simulink model "Lab8"  (R2022b)
settings: Solver=ode1  StartTime=0.0  StopTime=300  FixedStep=0.01  RelTol=1e-3
values from neighbouring files (symbols this model uses):
  Ap = 2.5    [Lab08.m]
  As = 0.1    [Lab08.m]
  fp = 0.2    [Lab08.m]
  fs = 0.015    [Lab08.m]
  Kp = 6    [Lab08.m]
  Ks = 1    [Lab08.m]
libraries: simulink x1, simulink_extras x1
settings Model: Creator=Wasif  LastModifiedBy=Wasif
settings DataIOCC: ReturnWorkspaceOutputs=off

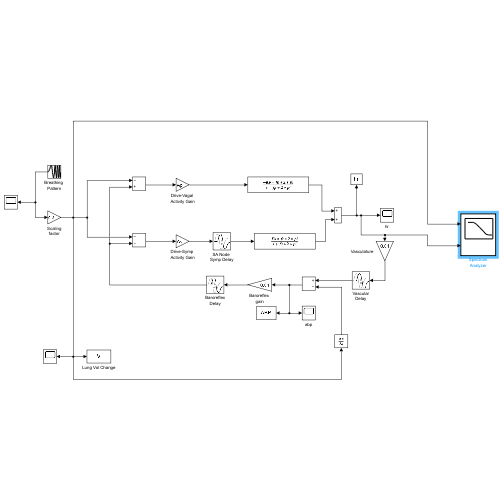
[thumbnail: Simulink's stored preview of the top-level diagram]
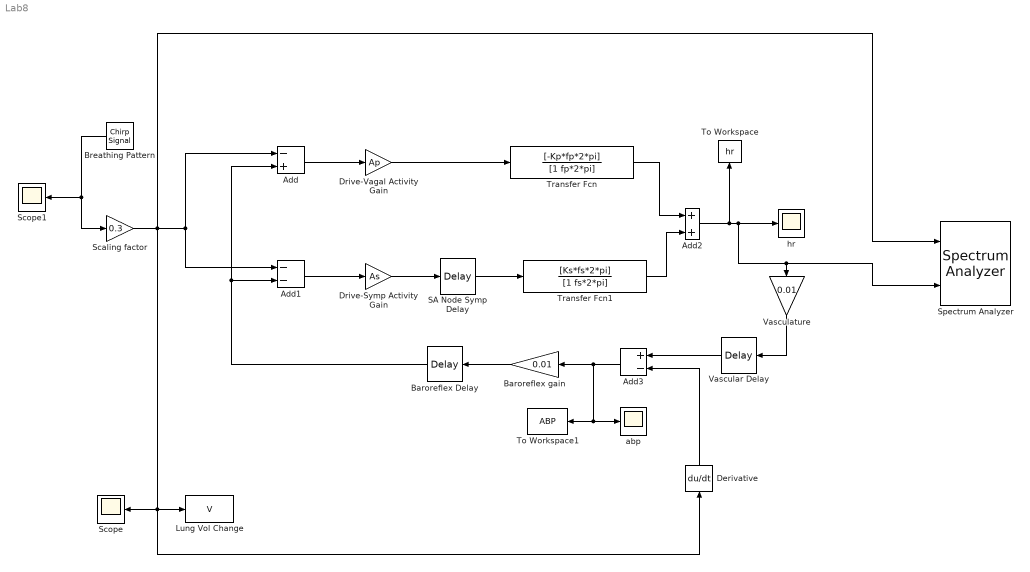
== system Lab8 ==
  Add : Sum  Inputs=-+
  Add1 : Sum  Inputs=--
  Add2 : Sum
  Add3 : Sum  Inputs=+-
  Baroreflex Delay : TransportDelay  DelayTime=0.3
  Baroreflex gain : Gain  Gain=0.01
  Breathing Pattern : simulink/Sources/Chirp Signal  f1=0.005  T=300  f2=0.5
  Derivative : Derivative
  Drive-Symp Activity Gain : Gain  Gain=As
  Drive-Vagal Activity Gain : Gain  Gain=Ap
  Lung Vol Change : ToWorkspace  VariableName=V  SampleTime=-1
  SA Node Symp Delay : TransportDelay  DelayTime=1.7
  Scaling factor : Gain  Gain=0.3
  Scope : Scope
  Scope1 : Scope
  Spectrum Analyzer : simulink_extras/Additional Sinks/Spectrum Analyzer  npts=256  fftpts=256  HowOften=64  sampleT=0.1
  To Workspace : ToWorkspace  VariableName=hr  SampleTime=-1
  To Workspace1 : ToWorkspace  VariableName=ABP  SampleTime=-1
  Transfer Fcn : TransferFcn  Numerator=[-Kp*fp*2*pi]  Denominator=[1 fp*2*pi]
  Transfer Fcn1 : TransferFcn  Numerator=[Ks*fs*2*pi]  Denominator=[1 fs*2*pi]
  Vascular Delay : TransportDelay  DelayTime=0.44
  Vasculature : Gain  Gain=0.01
  abp : Scope
  hr : Scope
  wires:
  Breathing Pattern/1 -> Scope1/1, Scaling factor/1
  Scaling factor/1 -> Derivative/1, Scope/1, Lung Vol Change/1, Spectrum Analyzer/1, Add/1, Add1/1
  Add/1 -> Drive-Vagal Activity Gain/1
  Add1/1 -> Drive-Symp Activity Gain/1
  Drive-Symp Activity Gain/1 -> SA Node Symp Delay/1
  Drive-Vagal Activity Gain/1 -> Transfer Fcn/1
  SA Node Symp Delay/1 -> Transfer Fcn1/1
  Transfer Fcn/1 -> Add2/1
  Transfer Fcn1/1 -> Add2/2
  Add2/1 -> To Workspace/1, Spectrum Analyzer/2, Vasculature/1, hr/1
  Vasculature/1 -> Vascular Delay/1
  Vascular Delay/1 -> Add3/1
  Add3/1 -> abp/1, To Workspace1/1, Baroreflex gain/1
  Baroreflex gain/1 -> Baroreflex Delay/1
  Baroreflex Delay/1 -> Add/2, Add1/2
  Derivative/1 -> Add3/2
